simulink model "lab_harmonic_mdl"  (R2023a)
settings: Solver=ode15s  StartTime=0.0  StopTime=5  RelTol=1e-3  EnableMultiTasking=on
values from neighbouring files (symbols this model uses):
  a = a_var(k)    [LAB2.m]    (also in relay.m = 15.5)
  b = %0.1f    [LAB2.m]    (also in q.m = 1; q_dot.m = 1; relay.m = 1)
  c = %0.1f', a, b, c)    [LAB2.m]    (also in q.m = 1; q_dot.m = 1; relay.m = 1)
  dzeta = 0.5    [LAB2.m]
  K1 = 25    [LAB2.m]
  omega = 5    [LAB2.m]
  omega_so = 8.31    [LAB2.m]
  T1 = 0.05    [LAB2.m]
settings Model: Creator=lobachev  LastModifiedBy=sonno
settings SolverCC: AlgebraicLoopSolver=TrustRegion  AutoInsertRateTranBlk=on
settings DataIOCC: SaveOutput=off  SaveTime=off
settings OptimizationCC: DefaultParameterBehavior=Inlined  InlineInvariantSignals=on  EnhancedBackFolding=on  PassReuseOutputArgsAs=Individual arguments  StateBitsets=on  DataBitsets=on  ZeroExternalMemoryAtStartup=off  ZeroInternalMemoryAtStartup=off  NoFixptDivByZeroProtection=on  LifeSpan=1  OptimizeBlockOrder=speed  DifferentSizesBufferReuse=on  EfficientTunableParamExpr=on
settings DebuggingCC: ParameterTunabilityLossMsg=error  UnconnectedInputMsg=warning  UnconnectedOutputMsg=warning  UnconnectedLineMsg=warning
settings HardwareCC: ProdBitPerPointer=32  ProdBitPerSizeT=32  ProdBitPerPtrDiffT=32  ProdLargestAtomicFloat=None  ProdIntDivRoundTo=Floor  ProdWordSize=32  ProdHWDeviceType=Generic->Custom
settings ModelReferenceCC: EnableRefExpFcnMdlSchedulingChecks=on
settings SFSimCC: MATLABDynamicMemAlloc=off
settings RTWCC: Description=Embedded Coder  SystemTargetFile=ert.tlc  TLCOptions=-p0  GenCodeOnly=on  TemplateMakefile=ert_default_tmf  GenerateReport=on  RTWVerbose=off  IncludeHyperlinkInReport=on  LaunchReport=on  DLArmComputeVersion=19.05
settings CodeAppCC: ForceParamTrailComments=on  IgnoreCustomStorageClasses=off  OperatorAnnotations=on  SimulinkDataObjDesc=on  SFDataObjDesc=on  CustomSymbolStrGlobalVar=rt$N$M  CustomSymbolStrType=$N$M  CustomSymbolStrFcn=$N$M$F  CustomSymbolStrMacro=$N$M  InsertBlockDesc=on
settings ERTTargetCC: TargetLangStandard=C99 (ISO)  CodeReplacementLibrary=ISO_C  GenerateSampleERTMain=on  IncludeMdlTerminateFcn=off  SuppressErrorStatus=on  SupportAbsoluteTime=off  PurelyIntegerCode=on  SupportNonFinite=off  SupportComplex=off  InlinedParameterPlacement=NonHierarchical  RootIOFormat=Structure reference  ERTCustomFileTemplate=example_file_process.tlc

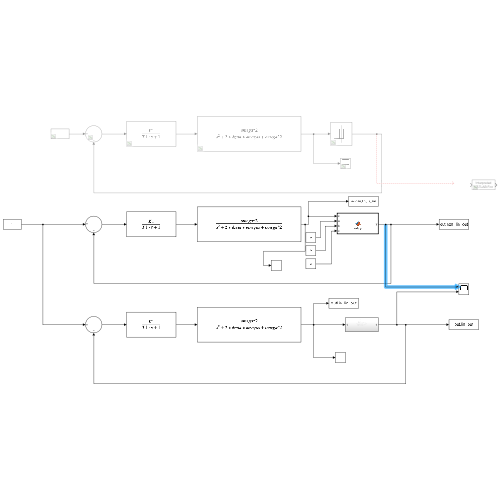
[thumbnail: Simulink's stored preview of the top-level diagram]
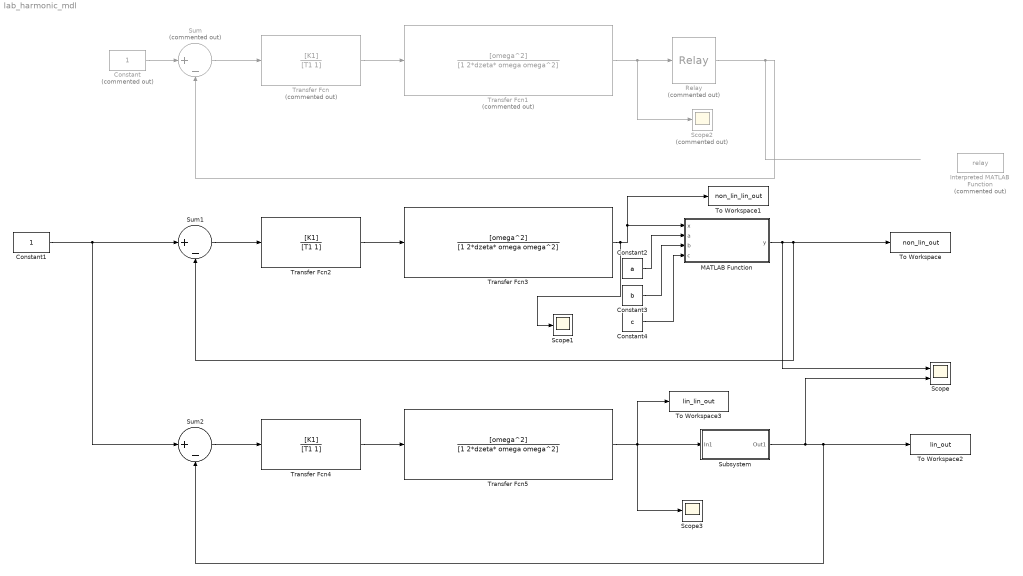
== system lab_harmonic_mdl ==
  Constant : Constant  Commented=on
  Constant1 : Constant
  Constant2 : Constant  Value=a
  Constant3 : Constant  Value=b
  Constant4 : Constant  Value=c
  Interpreted MATLAB Function : MATLABFcn  Commented=on  MATLABFcn=relay  OutputSignalType=real
  MATLAB Function : MATLAB Function  TreatAsAtomicUnit=on
  Relay : Relay  Commented=on  OnSwitchValue=b  OffSwitchValue=b  OnOutputValue=c  OffOutputValue=-c
  Scope : Scope  NumInputPorts=2
  Scope1 : Scope
  Scope2 : Scope  Commented=on
  Scope3 : Scope
  Subsystem : Subsystem
  Sum : Sum  Commented=on  Inputs=|+-
  Sum1 : Sum  Inputs=|+-
  Sum2 : Sum  Inputs=|+-
  To Workspace : ToWorkspace  VariableName=non_lin_out  SaveFormat=Structure With Time  SampleTime=-1
  To Workspace1 : ToWorkspace  VariableName=non_lin_lin_out  SaveFormat=Structure With Time  SampleTime=-1
  To Workspace2 : ToWorkspace  VariableName=lin_out  SaveFormat=Structure With Time  SampleTime=-1
  To Workspace3 : ToWorkspace  VariableName=lin_lin_out  SaveFormat=Structure With Time  SampleTime=-1
  Transfer Fcn : TransferFcn  Commented=on  Numerator=[K1]  Denominator=[T1 1]
  Transfer Fcn1 : TransferFcn  Commented=on  Numerator=[omega^2]  Denominator=[1 2*dzeta* omega omega^2]
  Transfer Fcn2 : TransferFcn  Numerator=[K1]  Denominator=[T1 1]
  Transfer Fcn3 : TransferFcn  Numerator=[omega^2]  Denominator=[1 2*dzeta* omega omega^2]
  Transfer Fcn4 : TransferFcn  Numerator=[K1]  Denominator=[T1 1]
  Transfer Fcn5 : TransferFcn  Numerator=[omega^2]  Denominator=[1 2*dzeta* omega omega^2]
  wires:
  Transfer Fcn/1 -> Transfer Fcn1/1
  Transfer Fcn1/1 -> Scope2/1, Relay/1
  Sum/1 -> Transfer Fcn/1
  Relay/1 -> Sum/2
  Constant/1 -> Sum/1
  MATLAB Function/1(y) -> Scope/1, To Workspace/1, Sum1/2
  Sum1/1 -> Transfer Fcn2/1
  Transfer Fcn2/1 -> Transfer Fcn3/1
  Transfer Fcn3/1 -> MATLAB Function/1(x), To Workspace1/1, Scope1/1
  Transfer Fcn4/1 -> Transfer Fcn5/1
  Sum2/1 -> Transfer Fcn4/1
  Subsystem/1(Out1) -> Scope/2, To Workspace2/1, Sum2/2
  Constant1/1 -> Sum2/1, Sum1/1
  Transfer Fcn5/1 -> Scope3/1, To Workspace3/1, Subsystem/1(In1)
  Constant2/1 -> MATLAB Function/2(a)
  Constant3/1 -> MATLAB Function/3(b)
  Constant4/1 -> MATLAB Function/4(c)

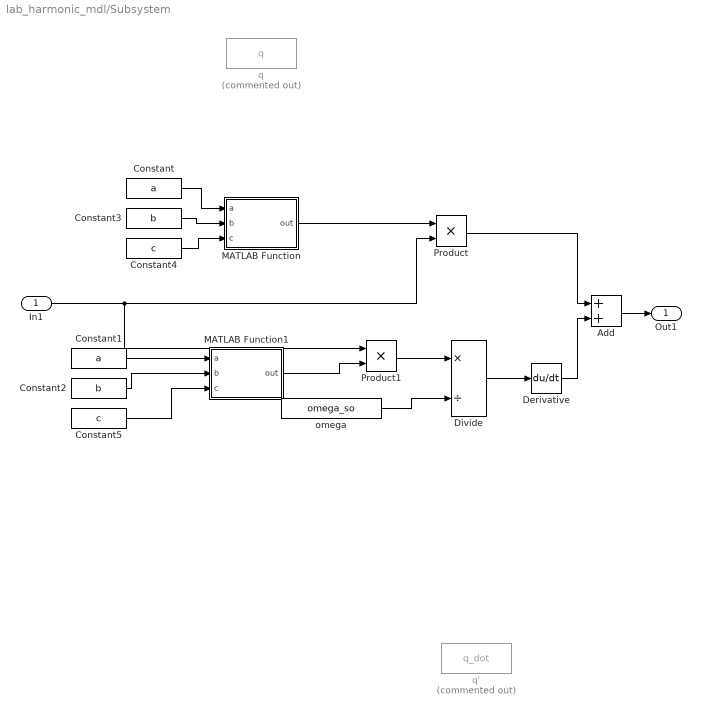
== system lab_harmonic_mdl/Subsystem ==
  In1 : Inport
  Add : Sum
  Constant : Constant  Value=a
  Constant1 : Constant  Value=a
  Constant2 : Constant  Value=b
  Constant3 : Constant  Value=b
  Constant4 : Constant  Value=c
  Constant5 : Constant  Value=c
  Derivative : Derivative  CoefficientInTFapproximation=0
  Divide : Product  Inputs=*/
  MATLAB Function : MATLAB Function  TreatAsAtomicUnit=on
  MATLAB Function1 : MATLAB Function  TreatAsAtomicUnit=on
  Product : Product
  Product1 : Product
  omega : Constant  Value=omega_so
  q : MATLABFcn  Commented=on  MATLABFcn=q
  q' : MATLABFcn  Commented=on  MATLABFcn=q_dot
  Out1 : Outport
  wires:
  In1/1 -> Product1/1, Product/2
  MATLAB Function/1(out) -> Product/1
  MATLAB Function1/1(out) -> Product1/2
  Product1/1 -> Divide/1
  omega/1 -> Divide/2
  Divide/1 -> Derivative/1
  Product/1 -> Add/1
  Derivative/1 -> Add/2
  Add/1 -> Out1/1
  Constant/1 -> MATLAB Function/1(a)
  Constant3/1 -> MATLAB Function/2(b)
  Constant4/1 -> MATLAB Function/3(c)
  Constant1/1 -> MATLAB Function1/1(a)
  Constant2/1 -> MATLAB Function1/2(b)
  Constant5/1 -> MATLAB Function1/3(c)

== matlab function lab_harmonic_mdl/Subsystem/MATLAB Function ==
  data: a input; out output; b input; c input
function out = q(a, b, c)

% a = 15.5;
% b = 1;
% c = 1;
out = 4*c/(pi * a) * sqrt(1 - (b/a)^2);

end

== matlab function lab_harmonic_mdl/MATLAB Function ==
  settings: updateMethod=DISCRETE
  data: x input; y output; a input; b input; c input
function y = relay(x, a, b, c) %

lower = -1;
upper = 1;

% a = 15.5;
% b = 1;
% c = 1;

persistent sts y_prev

if isempty(sts)
    
    sts = lower;
    y_prev = -1;
end

if (sts == upper) && (x <= -b)
    
    y = -c;
    sts = lower;
elseif (sts == lower) && (x >= b)
    
    y = c;
    sts = upper;
else
    
    y = y_prev;
end

y_prev = y;
end

== matlab function lab_harmonic_mdl/Subsystem/MATLAB Function1 ==
  data: a input; out output; b input; c input
function out = q_dot(a, b, c)

% a = 15.5;
% b = 1;
% c = 1;

if (a >= b)
    
    out = -4*c*b/(pi*a^2);
else
    
    out = 0;    
end

end
